simulink model "commblksgettingstarted"  (Simulink 5.0)
settings: Solver=ode45  SolverMode=SingleTasking  StartTime=0.0  StopTime=inf  RelTol=1e-3
libraries: dspbuff3 x2, commcnvcod2 x2, commchan2 x1, commdigbbndpm2 x1, commsource2 x1, commsink2 x1, commsrccod2 x1
Description:
  | Example described in Release 12.0 version of Communications Blockset User's Guide.
  | Similar to the Soft-Decision Decoding example described in Release 12.1 version.
settings Model: RequirementInfo=9  CovMetricSettings=d  Creator=mikem  LastModifiedBy=sramaswa  SaveState=on  SaveFormat=Structure  LimitDataPoints=off  IntegerOverflowMsg=none  ExtModeTrigMode=oneshot  ExtModeArmWhenConnect=off  BlockReductionOpt=off  BooleanDataType=off

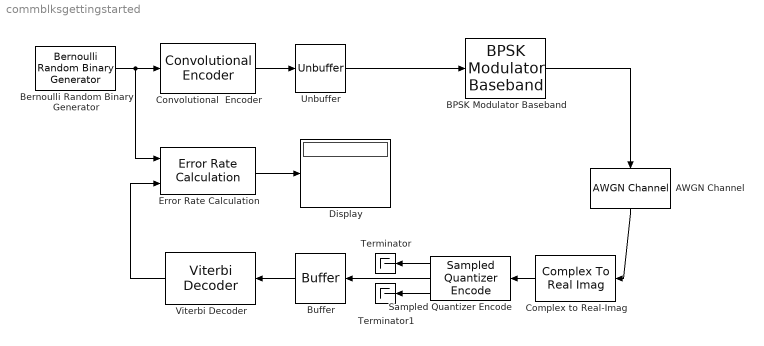
== system commblksgettingstarted ==
  AWGN Channel : commchan2/AWGN Channel  Orientation=down  seed=123456  noiseMode="Signal to noise ratio  (Es/No)"  EsNodB=-1  SNRdB=10  Ps=1  Tsym=.5  variance=1
  BPSK Modulator Baseband : commdigbbndpm2/BPSK Modulator Baseband  Ph=0  numSamp=1
  Bernoulli Random Binary Generator : commsource2/Bernoulli Random Binary Generator  P=0.5  seed=12345  Ts=1  frameBased=on  sampPerFrame=1  orient=off
  Buffer : dspbuff3/Buffer  Orientation=left  N=2  V=0  ic=0
  Complex to Real-Imag : ComplexToRealImag  Orientation=left  Output=Real
  Convolutional  Encoder : commcnvcod2/Convolutional Encoder  trellis=poly2trellis(7, [171 133])  reset=None
  Display : Display
      settings: Format=short
  Error Rate Calculation : commsink2/Error Rate Calculation  N=49  st_delay=0  cp_mode=Entire frame  subframe=[]  PMode=Port  WsName=ErrorVec  RsMode2=off  stop=off  numErr=100  maxBits=1e6
  Sampled Quantizer Encode : commsrccod2/Sampled Quantizer Encode  Orientation=left  partition=[-.75 -.5 -.25 0 .25 .5 .75]  codebook=[7 6 5 4 3 2 1 0]  n=1  sample_time=-1
  Terminator : Terminator
  Terminator1 : Terminator
  Unbuffer : dspbuff3/Unbuffer  ic=0
  Viterbi Decoder : commcnvcod2/Viterbi Decoder  Orientation=left  trellis=poly2trellis(7, [171 133])  dectype=Soft Decision  nsdecb=3  tbdepth=48  opmode=Continuous  reset=off
  wires:
  Convolutional  Encoder/1 -> Unbuffer/1
  Unbuffer/1 -> BPSK Modulator Baseband/1
  BPSK Modulator Baseband/1 -> AWGN Channel/1
  Bernoulli Random Binary Generator/1 -> Error Rate Calculation/1, Convolutional  Encoder/1
  Error Rate Calculation/1 -> Display/1
  Sampled Quantizer Encode/1 -> Terminator/1
  Sampled Quantizer Encode/3 -> Terminator1/1
  Buffer/1 -> Viterbi Decoder/1
  Viterbi Decoder/1 -> Error Rate Calculation/2
  Sampled Quantizer Encode/2 -> Buffer/1
  AWGN Channel/1 -> Complex to Real-Imag/1
  Complex to Real-Imag/1 -> Sampled Quantizer Encode/1
